simulink model "test"  (Simulink 7.1)
settings: Solver=ode45  StartTime=0.0  StopTime=10.0  RelTol=1e-3
settings Model: Creator=glaurent  LastModifiedBy=glaurent  ExtModeTrigMode=oneshot  ExtModeArmWhenConnect=off
settings DataIOCC: LimitDataPoints=off
settings OptimizationCC: BlockReduction=off  BooleanDataType=off
settings DebuggingCC: SaveWithParameterizedLinksMsg=none  SignalResolutionControl=TryResolveAllWithWarning  SolverPrmCheckMsg=none  MultiTaskDSMMsg=warning  MultiTaskCondExecSysMsg=none  StrictBusMsg=None
settings HardwareCC: TargetUnknown=on
settings RTWCC: IncludeERTFirstTime=on
settings GRTTargetCC: ModelReferenceCompliant=off  CompOptLevelCompliant=off  MatFileLogging=off

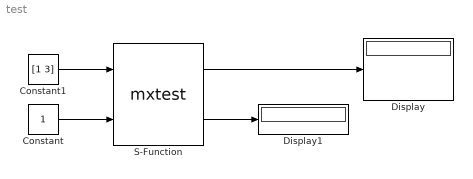
== system test ==
  Constant : Constant
  Constant1 : Constant  Value=[1 3]
  Display : Display
  Display1 : Display
  S-Function : S-Function  FunctionName=mxtest  Parameters=[10 20] 2 'testmat'  EnableBusSupport=off
  wires:
  Constant1/1 -> S-Function/1
  Constant/1 -> S-Function/2
  S-Function/1 -> Display/1
  S-Function/2 -> Display1/1
